simulink model "observer"  (R2024b)
settings: Solver=FixedStepAuto  StartTime=0.0  StopTime=Tend  FixedStep=0.0001  RelTol=1e-4
values from neighbouring files (symbols this model uses):
  b = 4.28e-6    (= 4.28e-06)    [setup.m]    (also in test.m)
  b_o_sf = wb_sf*J_z    (= 0.00185605293974)    [setup.m]
  J_z = 29.54e-6    (= 2.954e-05)    [setup.m]
  K_io_sf = wb_sf*b    (= 0.000268920331147)    [setup.m]
  Ts = 1e-4    (= 0.0001)    [setup.m]    (also in test.m = 0.001)
undefined symbols (not defined in the file or in its folder): DiscIntNeverNeededParam
settings Model: Creator=puroh  LastModifiedBy=tnoguchi
settings DataIOCC: SaveOutput=off  SaveTime=off
settings OptimizationCC: DefaultParameterBehavior=Inlined  EnhancedBackFolding=on  PassReuseOutputArgsAs=Individual arguments  ZeroExternalMemoryAtStartup=off  ZeroInternalMemoryAtStartup=off  OptimizeBlockOrder=speed  DifferentSizesBufferReuse=on  EfficientTunableParamExpr=on
settings DebuggingCC: ParameterTunabilityLossMsg=error  UnconnectedInputMsg=warning  UnconnectedOutputMsg=warning  UnconnectedLineMsg=warning
settings ModelReferenceCC: EnableRefExpFcnMdlSchedulingChecks=on
settings SFSimCC: MATLABDynamicMemAlloc=off
settings RTWCC: Description=Embedded Coder  SystemTargetFile=ert.tlc  TemplateMakefile=ert_default_tmf  GPUComputeCapability=3.5  DLArmComputeVersion=19.05
settings CodeAppCC: ForceParamTrailComments=on  IgnoreCustomStorageClasses=off  OperatorAnnotations=on  SimulinkDataObjDesc=on  SFDataObjDesc=on  InsertBlockDesc=on
settings ERTTargetCC: TargetLangStandard=C99 (ISO)  ERTCustomFileTemplate=example_file_process.tlc  DynamicArrayContainerType=coder::array
settings ConfigComp: CovBoundaryAbsTol=1.0e-5

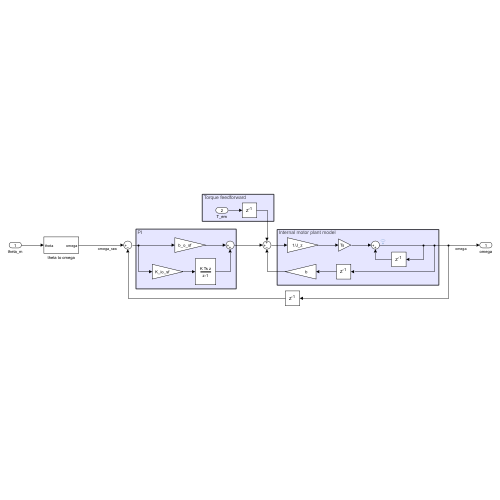
[thumbnail: Simulink's stored preview of the top-level diagram]
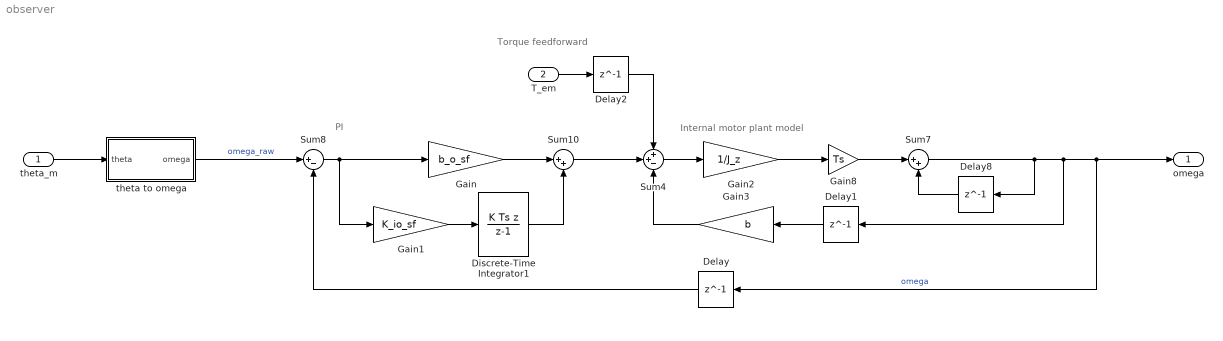
== system observer ==
  note: Torque feedforward
  note: PI
  note: Internal motor plant model
  theta_m : Inport  OutDataTypeStr=double  PortDimensions=1  SampleTime=[0.0001,0]
  T_em : Inport  Port=2  OutDataTypeStr=double  PortDimensions=1  SampleTime=[0.0001,0]
  Delay{,1..2,8} (4 alike) : Delay  DelayLength=1  InputProcessing=Columns as channels (frame based)
  Discrete-Time Integrator1 : DiscreteIntegrator  IntegratorMethod=Integration: Backward Euler  SampleTime=-1  ICPrevOutput=DiscIntNeverNeededParam  ICPrevScaledInput=DiscIntNeverNeededParam
  Gain : Gain  Gain=b_o_sf
  Gain1 : Gain  Gain=K_io_sf
  Gain2 : Gain  Gain=1/J_z
  Gain3 : Gain  Gain=b
  Gain8 : Gain  Gain=Ts
  Sum10 : Sum  Inputs=|++
  Sum4 : Sum  Inputs=++-
  Sum7 : Sum  Inputs=|++
  Sum8 : Sum  Inputs=|+-
  theta to omega : Subsystem
  omega : Outport  OutDataTypeStr=double  PortDimensions=1  SampleTime=[0.0001,0]
  wires:
  theta to omega/1(omega) -> Sum8/1  "omega_raw"
  Delay8/1 -> Sum7/2
  Sum8/1 -> Gain/1, Gain1/1
  Gain1/1 -> Discrete-Time Integrator1/1
  Delay/1 -> Sum8/2
  Delay2/1 -> Sum4/1
  Gain/1 -> Sum10/1
  T_em/1 -> Delay2/1
  Sum4/1 -> Gain2/1
  Gain8/1 -> Sum7/1
  Discrete-Time Integrator1/1 -> Sum10/2
  Sum7/1 -> Delay8/1, Delay1/1, Delay/1, omega/1  "omega"
  Sum10/1 -> Sum4/2
  theta_m/1 -> theta to omega/1(theta)
  Gain3/1 -> Sum4/3
  Delay1/1 -> Gain3/1
  Gain2/1 -> Gain8/1

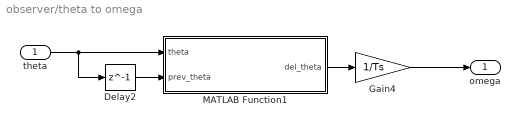
== system observer/theta to omega ==
  theta : Inport
  Delay2 : Delay  DelayLength=1  InputProcessing=Columns as channels (frame based)
  Gain4 : Gain  Gain=1/Ts
  MATLAB Function1 : MATLAB Function  TreatAsAtomicUnit=on
  omega : Outport
  wires:
  Gain4/1 -> omega/1
  MATLAB Function1/1(del_theta) -> Gain4/1
  Delay2/1 -> MATLAB Function1/2(prev_theta)
  theta/1 -> Delay2/1, MATLAB Function1/1(theta)

== matlab function observer/theta to omega/MATLAB Function1 ==
  data: theta input; del_theta output; prev_theta input
function del_theta = delta_theta(theta, prev_theta)

    % check if prev_theta exist before using to prevent error in 1st iteration 
    del_theta = theta - prev_theta;

    % prevent jumps in speed during 2pi to 0 transitions 
    while del_theta > pi
        del_theta = del_theta - 2*pi;
    end

    while del_theta < -pi
        del_theta = del_theta + 2*pi;
    end
    
end
